simulink model "neural_30102019"  (R2018b)
settings: Solver=VariableStepAuto  StartTime=0.0  StopTime=10.0  RelTol=1e-3
libraries: neural x206
(part 5 of 5)

== system neural_30102019/NARX Neural Network/Layer 2/Delays 1 ==
  "p{2}" : Inport  PortDimensions=100  SampleTime=1
      mask Display: e = 0.06;c1 = [120 230 180]/255;c2 = ([120 230 180]+0)/(256+128);c3 = ([120 230 180]+128)/(256+128);patch([0 1 1 0],[0 0 1 1],c1);patch([0 1 1 1-e 1-e 0+e],[0 0 1 1-e 0+e 0+e],c2);patch([0 0 1 1-e 0+e 0+e],[0 1 1 1-e 1-e 0+e],c3);plot([0 1 1 0 0],[0 0 1 1 0]);
  mux : Mux  Inputs=1
      mask Display: e = 0.06;c1 = [120 150 230]/255;c2 = ([120 150 230]+0)/383;c3 = ([120 150 230]+128)/383;patch([0 1 1 0],[0 0 1 1],c1);patch([0 1 1 1-e 1-e 0+e],[0 0 1 1-e 0+e 0+e],c2);patch([0 0 1 1-e 0+e 0+e],[0 1 1 1-e 1-e 0+e],c3);plot([0 1 1 0 0],[0 0 1 1 0]);disp('Mux')
  "pd{2,1}" : Outport
      mask Display: e = 0.06;c1 = [120 230 180]/255;c2 = ([120 230 180]+0)/(256+128);c3 = ([120 230 180]+128)/(256+128);patch([0 1 1 0],[0 0 1 1],c1);patch([0 1 1 1-e 1-e 0+e],[0 0 1 1-e 0+e 0+e],c2);patch([0 0 1 1-e 0+e 0+e],[0 1 1 1-e 1-e 0+e],c3);plot([0 1 1 0 0],[0 0 1 1 0]);
  wires:
  "p{2}"/1 -> mux/1
  mux/1 -> "pd{2,1}"/1

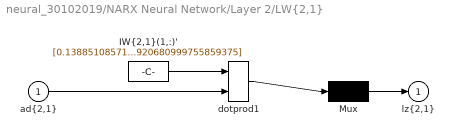
== system neural_30102019/NARX Neural Network/Layer 2/LW{2,1} ==
  "ad{2,1}" : Inport  PortDimensions=100  SampleTime=1
      mask Display: e = 0.06;c1 = [120 230 180]/255;c2 = ([120 230 180]+0)/(256+128);c3 = ([120 230 180]+128)/(256+128);patch([0 1 1 0],[0 0 1 1],c1);patch([0 1 1 1-e 1-e 0+e],[0 0 1 1-e 0+e 0+e],c2);patch([0 0 1 1-e 0+e 0+e],[0 1 1 1-e 1-e 0+e],c3);plot([0 1 1 0 0],[0 0 1 1 0]);
  "IW{2,1}(1,:)'" : Constant  Value=[0.13885108571050164272264737519435584545135498046875;0.1319576902494865866533046983022359199821949005126953125;-0.1339124165244286179810018211355782113969326019287109375;0.1209746516766650181740061498203431256115436553955078125;0.139124100720394661134804437097045592963695526123046875;-0.12182901298259811440072297727965633384883403778076171875;0.13671949802957772401867941880482248961925506591796875;0.142081401435798782006969531721551902592182159423828125;-0.48048673255083096389483898747130297124385833740234375;-0.117254681702811003329856021082377992570400238037109375;-0.44503301407462292349492827270296402275562286376953125;-0.13480623823943338468467345592216588556766510009765625;0.05102987541254842829285820471341139636933803558349609375;-0.1319345016580732998789926568861119449138641357421875;0.1404694130984556199592816483345814049243927001953125;-0.9089322368806669327767622235114686191082000732421875;0.14799379564557912924982474578428082168102264404296875;-0.143401781312660625555821525267674587666988372802734375;-0.1460679808448646366247913874758523888885974884033203125;-0.10362538797494662279330412957278895191848278045654296875;-0.144443203343128490079294579118140973150730133056640625;0.12893474853649411482336972767370752990245819091796875;0.132958464892300620707743519233190454542636871337890625;-0.779178085364024664016824317513965070247650146484375;0.98198769711140443394725707548786886036396026611328125;0.1257762387592722685969448548348736949265003204345703125;0.490972262403762516047578401412465609610080718994140625;-0.683432353784890533887619312736205756664276123046875;-0.86279162447850843431496059565688483417034149169921875;-1.269939959784590843838714135927148163318634033203125;-0.1427610506987519733979041802740539424121379852294921875;-0.97243343595598485951114753333968110382556915283203125;-0.1459060001526555350181979520129971206188201904296875;-0.56649326152753598506706111948005855083465576171875;0.7640225281487678099523463970399461686611175537109375;0.1350235699866686733816578680489328689873218536376953125;0.83983301801207710379770787767483852803707122802734375;0.5131888426150108539758321057888679206371307373046875;0.1356007630481496917251860168107668869197368621826171875;-0.92572045939459091101753074326552450656890869140625;-0.7836603153729868598276198099483735859394073486328125;0.1353692511678338539216071012560860253870487213134765625;0.147152511128743224144699297539773397147655487060546875;0.58712063785426649165088974768877960741519927978515625;-0.94974897396396773530113932793028652667999267578125;-0.83776800455559141678207879522233270108699798583984375;0.66894589197435772032207523807301186025142669677734375;-0.6570385243840937139481184203759767115116119384765625;-0.1371642241527550876156738013378344476222991943359375;-0.47906515283798400961501329220482148230075836181640625;-0.8212949803184692587620929771219380199909210205078125;-0.851871004836697753859198201098479330539703369140625;0.7024989943937722802758116813492961227893829345703125;0.77111915631099936518921822425909340381622314453125;0.1511185250188256390391217109936405904591083526611328125;0.1385649368115679791468863868431071750819683074951171875;-0.80833267500007466299649649954517371952533721923828125;0.51997543572602544781346978197689168155193328857421875;-0.66568547266070365875378911368898116052150726318359375;-0.11152945340408974839174760518289986066520214080810546875;-0.75548577843816044907754303494584746658802032470703125;0.118951713642144463189964653793140314519405364990234375;-0.491183075052584128261656815084279514849185943603515625;-0.685090054490654853935893697780556976795196533203125;-0.61506916564345714970585277114878408610820770263671875;-0.55808529954554153551526951559935696423053741455078125;0.56875779089223266193897643461241386830806732177734375;0.6527447594171194023005000417470000684261322021484375;-0.75030853128965413478823620607727207243442535400390625;-0.12368346137965517683721117236927966587245464324951171875 ...(+1708 chars)]
      mask Display: e = 0.06;c1 = [120 150 230]/255;c2 = ([120 150 230]+0)/383;c3 = ([120 150 230]+128)/383;patch([0 1 1 0],[0 0 1 1],c1);patch([0 1 1 1-e 1-e 0+e],[0 0 1 1-e 0+e 0+e],c2);patch([0 0 1 1-e 0+e 0+e],[0 1 1 1-e 1-e 0+e],c3);plot([0 1 1 0 0],[0 0 1 1 0]);disp('weights');
  Mux : Mux  Inputs=1
      mask Display: e = 0.06;c1 = [120 150 230]/255;c2 = ([120 150 230]+0)/383;c3 = ([120 150 230]+128)/383;patch([0 1 1 0],[0 0 1 1],c1);patch([0 1 1 1-e 1-e 0+e],[0 0 1 1-e 0+e 0+e],c2);patch([0 0 1 1-e 0+e 0+e],[0 1 1 1-e 1-e 0+e],c3);plot([0 1 1 0 0],[0 0 1 1 0]);disp('Mux');
  dotprod1 : neural/Weight Functions/dotprod
  "lz{2,1}" : Outport
      mask Display: e = 0.06;c1 = [120 230 180]/255;c2 = ([120 230 180]+0)/(256+128);c3 = ([120 230 180]+128)/(256+128);patch([0 1 1 0],[0 0 1 1],c1);patch([0 1 1 1-e 1-e 0+e],[0 0 1 1-e 0+e 0+e],c2);patch([0 0 1 1-e 0+e 0+e],[0 1 1 1-e 1-e 0+e],c3);plot([0 1 1 0 0],[0 0 1 1 0]);
  wires:
  "IW{2,1}(1,:)'"/1 -> dotprod1/1
  "ad{2,1}"/1 -> dotprod1/2
  dotprod1/1 -> Mux/1
  Mux/1 -> "lz{2,1}"/1
